simulink model "kurs_UV"  (R2023a)
settings: Solver=VariableStepAuto  StartTime=0.0  StopTime=10.0  RelTol=1e-3
values from neighbouring files (symbols this model uses):
  a = 0.4    [parameters_UV.m]
  alpha = pi /4    (= 0.785398163397)    [parameters_UV.m]
  Cwy1 = 259    [parameters_UV.m]
  Cwy2 = 26    [parameters_UV.m]
  firstPsi = 0 * pi / 180    (= 0)    [parameters_UV.m]
  Jy = 351    [parameters_UV.m]
  K1 = 44.8    [parameters_UV.m]
  K1Analytically = Kpsi / Kw    [parameters_UV.m]
  K2 = 27.6    [parameters_UV.m]
  K2Analytically = (((Tuv + Tdv)/(2*epsw*sqrt(Tdv*Tuv)))^2 - 1) /      (KdvTotal * Kuv)    [parameters_UV.m]
  Kdv = 100    [parameters_UV.m]
  lambda55 = 344    [parameters_UV.m]
  Mout = 0    [parameters_UV.m]
  Tdv = 0.15    [parameters_UV.m]
  Umax = 10    [parameters_UV.m]
libraries: simulink x1
settings Model: Creator=vilin  LastModifiedBy=vilin

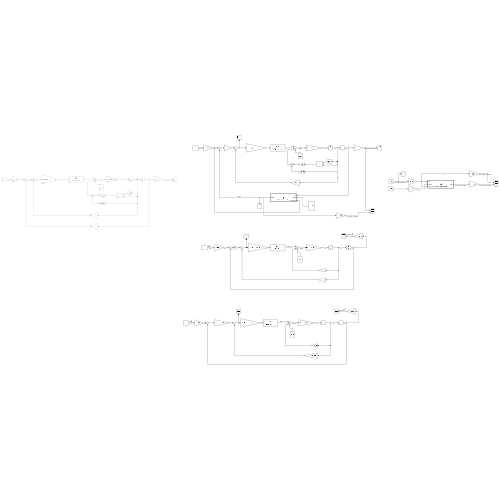
[thumbnail: Simulink's stored preview of the top-level diagram]
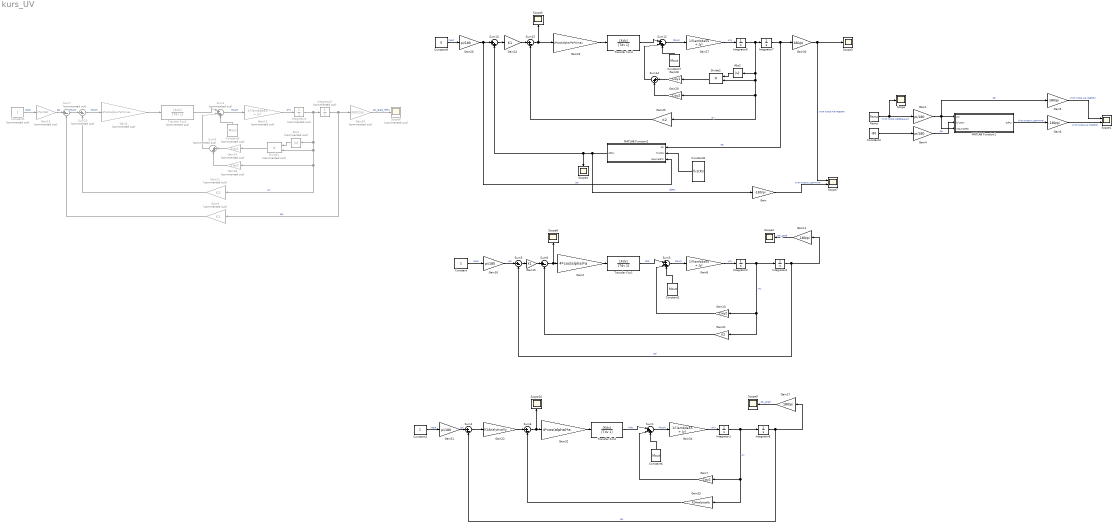
== system kurs_UV ==
  Abs1 : Abs  Commented=on  SaturateOnIntegerOverflow=off
  Abs2 : Abs  SaturateOnIntegerOverflow=off
  Constant : Constant
  Constant1 : Constant  Commented=on
  Constant2 : Constant  Value=Mout
  Constant3 : Constant
  Constant4 : Constant  Value=-80
  Constant5 : Constant  Commented=on  Value=Mout
  Constant6 : Constant  Value=Mout
  Constant7 : Constant  Value=Mout
  Constant8 : Constant  Value=firstPsi
  Constant9 : Constant  Value=0
  Divide1 : Product  Commented=on  Inputs=**
  Divide2 : Product  Inputs=**
  Gain : Gain  Gain=-180/pi
  Gain{1,4,16,26,31} (5 alike) : Gain  Gain=pi/180
  Gain10 : Gain  Gain=Cwy2
  Gain{5,11,17,30} (4 alike) : Gain  Gain=180/pi
  Gain12 : Gain  Commented=on  Gain=K2
  Gain13 : Gain  Commented=on  Gain=1/(lambda55 + Jy)
  Gain14 : Gain  Commented=on  Gain=Cwy1
  Gain15 : Gain  Gain=K1
  Gain18 : Gain  Commented=on  Gain=Cwy2
  Gain19 : Gain  Commented=on  Gain=2*pi/360
  Gain2 : Gain  Gain=4*cos(alpha)*a
  Gain20 : Gain  Commented=on  Gain=360/2/pi
  Gain21 : Gain  Gain=K2
  Gain22 : Gain  Gain=K1Analytically
  Gain23 : Gain  Gain=4*cos(alpha)*a*Umax
  Gain24 : Gain  Gain=K1
  Gain25 : Gain  Gain=K2
  Gain27 : Gain  Gain=1/(lambda55 + Jy)
  Gain28 : Gain  Gain=Cwy1
  Gain29 : Gain  Gain=Cwy2
  Gain3 : Gain  Commented=on  Gain=4*cos(alpha)*a*Umax
  Gain32 : Gain  Gain=4*cos(alpha)*a
  Gain33 : Gain  Gain=K2Analytically
  Gain34 : Gain  Gain=1/(lambda55 + Jy)
  Gain6 : Gain  Gain=-180/pi
  Gain7 : Gain  Gain=Cwy2
  Gain8 : Gain  Gain=1/(lambda55 + Jy)
  Gain9 : Gain  Commented=on  Gain=K1
  Integrator{1..3,6,8} (5 alike) : Integrator
  Integrator4 : Integrator  Commented=on
  Integrator5 : Integrator  Commented=on
  Integrator7 : Integrator  InitialCondition=firstPsi
  MATLAB Function1 : MATLAB Function  TreatAsAtomicUnit=on
  MATLAB Function2 : MATLAB Function  TreatAsAtomicUnit=on
  Ramp : simulink/Sources/Ramp  slope=10  start=0  InitialOutput=-80
  Scope{,2..5,8..10} (8 alike) : Scope
  Scope1 : Scope  NumInputPorts=2
  Scope6 : Scope  Commented=on
  Scope7 : Scope  NumInputPorts=2
  Sum1 : Sum  Inputs=|+-+
  Sum10 : Sum  Commented=on  Inputs=|+-
  Sum12 : Sum  Inputs=|+-+
  Sum13 : Sum  Inputs=|++
  Sum14 : Sum  Inputs=|++
  Sum{2,5..6,8,15} (5 alike) : Sum  Inputs=|+-
  Sum3 : Sum  Inputs=|+-+
  Sum4 : Sum  Commented=on  Inputs=|+-+
  Sum7 : Sum  Commented=on  Inputs=|+-
  Sum9 : Sum  Commented=on  Inputs=|++
  Transfer Fcn1 : TransferFcn  Numerator=[Kdv]  Denominator=[Tdv 1]
  Transfer Fcn2 : TransferFcn  Numerator=[Kdv]  Denominator=[Tdv 1]
  Transfer Fcn3 : TransferFcn  Commented=on  Numerator=[Kdv]  Denominator=[Tdv 1]
  Transfer Fcn4 : TransferFcn  Numerator=[Kdv]  Denominator=[Tdv 1]
  wires:
  Gain11/1 -> Scope2/1  "psi_grad"
  Sum3/1 -> Gain8/1  "Msum"
  Gain16/1 -> Sum5/1  "psi"
  Gain21/1 -> Sum8/2
  Gain10/1 -> Sum3/2
  Constant/1 -> Gain16/1  "input"
  Gain8/1 -> Integrator2/1  "w*y"
  Transfer Fcn1/1 -> Sum3/1  "Mdv"
  Integrator2/1 -> Integrator3/1, Gain21/1, Gain10/1  "wy"
  Integrator3/1 -> Gain11/1, Sum5/2  "psi"
  Sum8/1 -> Scope8/1, Gain2/1
  Constant2/1 -> Sum3/3
  Gain2/1 -> Transfer Fcn1/1
  Gain20/1 -> Scope6/1  "psi_grad_nelin"
  Integrator4/1 -> Abs1/1, Divide1/2, Gain18/1, Gain12/1, Integrator5/1  "wy"
  Gain14/1 -> Sum9/1
  Gain13/1 -> Integrator4/1  "w*y"
  Gain3/1 -> Transfer Fcn3/1
  Constant5/1 -> Sum4/3
  Sum4/1 -> Gain13/1  "Msum"
  Transfer Fcn3/1 -> Sum4/1
  Abs1/1 -> Divide1/1
  Sum10/1 -> Gain3/1  "Msum"
  Sum9/1 -> Sum4/2
  Integrator5/1 -> Gain9/1, Gain20/1  "psi"
  Divide1/1 -> Gain14/1
  Gain12/1 -> Sum10/2
  Gain18/1 -> Sum9/2
  Gain9/1 -> Sum7/2
  Constant1/1 -> Gain19/1  "input"
  Gain19/1 -> Sum7/1  "psi"
  Sum7/1 -> Sum10/1  "Msum"
  Gain26/1 -> MATLAB Function2/3(requiredPsi), Sum13/1  "psi"
  Constant9/1 -> Gain26/1  "input"
  Constant8/1 -> MATLAB Function2/2(firstPsi)
  Gain23/1 -> Transfer Fcn4/1
  Gain30/1 -> Scope7/1, Scope3/1  "угол курса на модели"
  Transfer Fcn4/1 -> Sum12/1
  Constant7/1 -> Sum12/3
  Sum15/1 -> Scope5/1, Gain23/1
  Gain27/1 -> Integrator6/1  "w*y"
  Gain25/1 -> Sum15/2
  Gain28/1 -> Sum14/1
  Divide2/1 -> Gain28/1
  Abs2/1 -> Divide2/1
  Integrator6/1 -> Abs2/1, Divide2/2, Gain29/1, Gain25/1, Integrator7/1  "wy"
  Sum14/1 -> Sum12/2
  Sum12/1 -> Gain27/1  "Msum"
  MATLAB Function2/1(difPsi) -> Gain/1, Sum13/2, Scope4/1  "difPsi"
  Gain29/1 -> Sum14/2
  Integrator7/1 -> MATLAB Function2/1(psi), Gain30/1  "psi"
  Sum13/1 -> Gain24/1
  Gain24/1 -> Sum15/1
  Sum5/1 -> Gain15/1
  Gain15/1 -> Sum8/1
  Gain/1 -> Scope7/2  "угол курса с датчика"
  Ramp/1 -> Scope/1, Gain1/1  "Угол курса идеальный"
  MATLAB Function1/1(difPsi) -> Gain6/1  "Угол курса с датчика"
  Constant4/1 -> Gain4/1
  Gain1/1 -> MATLAB Function1/3(requiredPsi), Gain5/1, MATLAB Function1/1(psi)  "psi"
  Gain4/1 -> MATLAB Function1/2(firstPsi)  "psi"
  Gain5/1 -> Scope1/1  "угол курса на модели"
  Gain6/1 -> Scope1/2  "угол курса на модели"
  Gain33/1 -> Sum6/2
  Integrator1/1 -> Integrator8/1, Gain33/1, Gain7/1  "wy"
  Gain17/1 -> Scope9/1  "psi_grad"
  Constant3/1 -> Gain31/1  "input"
  Sum1/1 -> Gain34/1  "Msum"
  Gain32/1 -> Transfer Fcn2/1
  Gain34/1 -> Integrator1/1  "w*y"
  Integrator8/1 -> Gain17/1, Sum2/2  "psi"
  Gain7/1 -> Sum1/2
  Gain31/1 -> Sum2/1  "psi"
  Sum6/1 -> Scope10/1, Gain32/1
  Constant6/1 -> Sum1/3
  Gain22/1 -> Sum6/1
  Sum2/1 -> Gain22/1
  Transfer Fcn2/1 -> Sum1/1  "Mdv"

== matlab function kurs_UV/MATLAB Function1 ==
  settings: updateMethod=DISCRETE  sampleTime=0.1
  data: psi input; difPsi output; firstPsi input; requiredPsi input
function difPsi  = ...
    calc_dif_psi_realtime(psi, firstPsi, requiredPsi)
coder.extrinsic('dbscan');

minAngleRotate = -180;
maxAngleRotate = 180;
stepAngleRotate = 0.5;

persistent isFirstIteration  prevDifPsi  rotatedImages maxDif;
if isempty(isFirstIteration)
    imageFileName = ('./test1_0.jpg');

    rotatedImages = generate_array_rotated_image(...
    imageFileName, minAngleRotate, maxAngleRotate, stepAngleRotate);

    psi = firstPsi;
    maxDif = 8 * pi / 180;

end

cannySigma = 3;
cannyThreshold = [];
houghParams = struct('threshold', 0.5, 'peaks', 4, 'FillGap', 3, 'MinLength', 5);
epsDbscan = 0.25;

curPsi = psi * 180 / pi - 3.75;
if curPsi > maxAngleRotate
    curPsi = maxAngleRotate;
end

if curPsi < minAngleRotate
    curPsi = minAngleRotate;
end

if curPsi < -2
    curPsi = curPsi; 
end

curImage = double(squeeze(rotatedImages(...
    round((curPsi- minAngleRotate)/stepAngleRotate)  + 1, :, :, :))) / 255;

requiredPsi = requiredPsi / 180 * pi;

difPsi = calc_dif_psi( ...
   requiredPsi, curImage, cannySigma, cannyThreshold, houghParams, epsDbscan);

if isempty(isFirstIteration)
    prevDifPsi = difPsi;
    isFirstIteration = 1;
end

if abs(difPsi - prevDifPsi) > maxDif
    difPsi = prevDifPsi;
    maxDif = maxDif * 1.1;

    return
end

maxDif = 8 * pi / 180;

prevDifPsi = difPsi;

== matlab function kurs_UV/MATLAB Function2 ==
  settings: updateMethod=DISCRETE  sampleTime=0.1
  data: psi input; difPsi output; firstPsi input; requiredPsi input
function difPsi  = ...
    calc_dif_psi_realtime(psi, firstPsi, requiredPsi)
coder.extrinsic('dbscan');

minAngleRotate = -180;
maxAngleRotate = 180;
stepAngleRotate = 0.5;

persistent isFirstIteration  prevDifPsi  rotatedImages maxDif;
if isempty(isFirstIteration)
    imageFileName = ('./test1_0.jpg');

    rotatedImages = generate_array_rotated_image(...
    imageFileName, minAngleRotate, maxAngleRotate, stepAngleRotate);

    psi = firstPsi;
    maxDif = 15 * pi / 180;

end

cannySigma = 3;
cannyThreshold = [];
houghParams = struct('threshold', 0.5, 'peaks', 4, 'FillGap', 3, 'MinLength', 5);
epsDbscan = 0.25;

curPsi = psi * 180 / pi - 3.75;
if curPsi > maxAngleRotate
    curPsi = maxAngleRotate;
end

if curPsi < minAngleRotate
    curPsi = minAngleRotate;
end

if curPsi < -2
    curPsi = curPsi; 
end

curImage = double(squeeze(rotatedImages(...
    round((curPsi- minAngleRotate)/stepAngleRotate)  + 1, :, :, :))) / 255;

requiredPsi = requiredPsi / 180 * pi;

difPsi = calc_dif_psi( ...
   requiredPsi, curImage, cannySigma, cannyThreshold, houghParams, epsDbscan);

if isempty(isFirstIteration)
    prevDifPsi = difPsi;
    isFirstIteration = 1;
end

if abs(difPsi - prevDifPsi) > maxDif
    difPsi = prevDifPsi;
    maxDif = maxDif * 1.1;

    return
end

maxDif = 15 * pi / 180;

prevDifPsi = difPsi;
